simulink subsystem "HI_VectorBox"  (R2019b)
settings: Solver=VariableStepAuto  StartTime=0.0  StopTime=10.0  RelTol=1e-3
undefined symbols (not defined in the file): motor1PWM, motor2PWM, motorControlMode, motorEnable, motorPosCommand_deg, motorPWMFreq, throttlePosInputMode
libraries: canmsglib x1, c280xlib x1
settings Model: Creator=Nick  LastModifiedBy=Nick

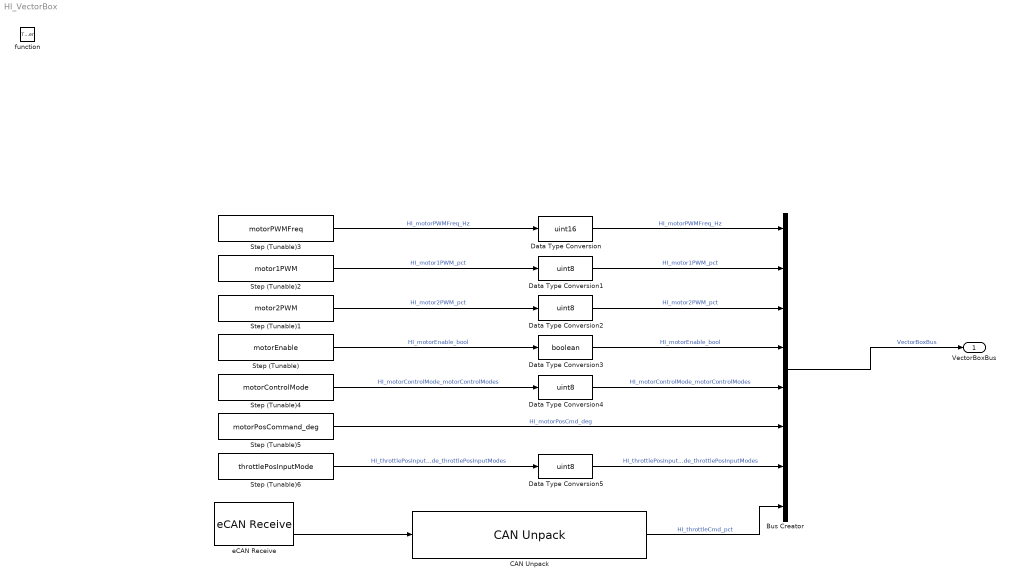
== system HI_VectorBox ==
  function : TriggerPort  TriggerType=function-call  VariantControl=Variant
  Bus Creator : BusCreator  Inputs=8
  CAN Unpack : canmsglib/CAN Unpack  CANdbFile=C:\Git\ETC-Development\DBCs\etc_benchTest.dbc  MsgList=VBOX_cmd1  MsgName=VBOX_cmd1  MsgIDType=Standard (11-bit identifier)  MsgIdentifier=500  MsgLength=2  SignalInfo={'VBOX_throttleCmd','0','16','LE','signed','Standard','0','0.01','0','-327.68','327.67'}  IDPort=off  TimestampPort=off  ErrorPort=off  RemotePort=off  LengthPort=off  StatusPort=off  ApplyMinMax=off
      settings: SourceProductName=Vehicle Network Toolbox  SourceProductBaseCode=VN  DataFormat=CANdb specified signals
  Data Type Conversion : DataTypeConversion  OutDataTypeStr=uint16
  Data Type Conversion{1..2,4..5} (4 alike) : DataTypeConversion  OutDataTypeStr=uint8
  Data Type Conversion3 : DataTypeConversion  OutDataTypeStr=boolean
  Step (Tunable) : Constant  Value=motorEnable  VectorParams1D=off  SampleTime=-1
  Step (Tunable)1 : Constant  Value=motor2PWM  VectorParams1D=off  SampleTime=-1
  Step (Tunable)2 : Constant  Value=motor1PWM  VectorParams1D=off  SampleTime=-1
  Step (Tunable)3 : Constant  Value=motorPWMFreq  VectorParams1D=off  SampleTime=-1
  Step (Tunable)4 : Constant  Value=motorControlMode  VectorParams1D=off  SampleTime=-1
  Step (Tunable)5 : Constant  Value=motorPosCommand_deg  VectorParams1D=off  SampleTime=-1
  Step (Tunable)6 : Constant  Value=throttlePosInputMode  VectorParams1D=off  SampleTime=-1
  eCAN Receive : c280xlib/eCAN Receive  chipFamily=C280x  useModule=eCAN_A  mailboxNo=11  messageID=500  messageType=Standard (11-bit identifier)  sampleTime=-1  dataType=CAN_MESSAGE_TYPE  initValue=0  outputMessageLength=off  outputMessageTimeStamp=off  postInterrupt=off  interruptLine=0
      settings: SourceProductName=Embedded Coder Support Package for Texas Instruments C2000 Processors  SourceProductBaseCode=TIC2000
  VectorBoxBus : Outport
  wires:
  Bus Creator/1 -> VectorBoxBus/1  "VectorBoxBus"
  Step (Tunable)3/1 -> Data Type Conversion/1  "HI_motorPWMFreq_Hz"
  Step (Tunable)2/1 -> Data Type Conversion1/1  "HI_motor1PWM_pct"
  Data Type Conversion1/1 -> Bus Creator/2  "HI_motor1PWM_pct"
  Data Type Conversion2/1 -> Bus Creator/3  "HI_motor2PWM_pct"
  Step (Tunable)1/1 -> Data Type Conversion2/1  "HI_motor2PWM_pct"
  Data Type Conversion3/1 -> Bus Creator/4  "HI_motorEnable_bool"
  Data Type Conversion/1 -> Bus Creator/1  "HI_motorPWMFreq_Hz"
  Step (Tunable)/1 -> Data Type Conversion3/1  "HI_motorEnable_bool"
  Step (Tunable)4/1 -> Data Type Conversion4/1  "HI_motorControlMode_motorControlModes"
  Data Type Conversion4/1 -> Bus Creator/5  "HI_motorControlMode_motorControlModes"
  Step (Tunable)5/1 -> Bus Creator/6  "HI_motorPosCmd_deg"
  eCAN Receive/2 -> CAN Unpack/1
  CAN Unpack/1 -> Bus Creator/8  "HI_throttleCmd_pct"
  Step (Tunable)6/1 -> Data Type Conversion5/1  "HI_throttlePosInputMode_throttlePosInputModes"
  Data Type Conversion5/1 -> Bus Creator/7  "HI_throttlePosInputMode_throttlePosInputModes"
